simulink model "roll_controller"  (R2021b)
settings: Solver=VariableStepAuto  StartTime=0.0  StopTime=10.0  RelTol=1e-3
settings Model: Creator=aoa  LastModifiedBy=aoa

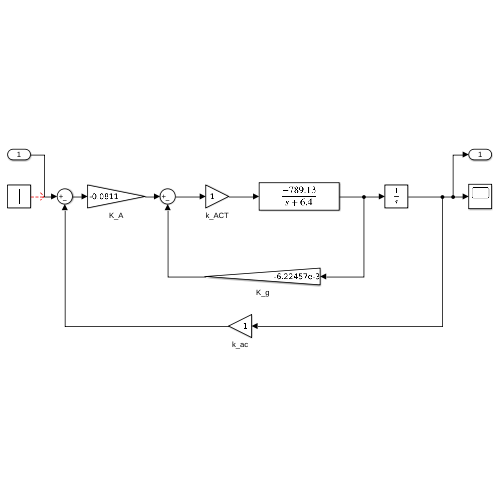
[thumbnail: Simulink's stored preview of the top-level diagram]
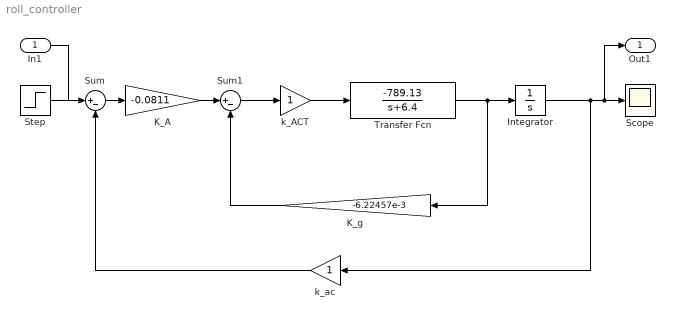
== system roll_controller ==
  In1 : Inport
  Integrator : Integrator
  K_A : Gain  Gain=-0.0811
  K_g : Gain  Gain=-6.22457e-3
  Scope : Scope
  Step : Step  SampleTime=0
  Sum : Sum  Inputs=|+-
  Sum1 : Sum  Inputs=|+-
  Transfer Fcn : TransferFcn  Numerator=[-789.13]  Denominator=[1 6.4]
  k_ACT : Gain
  k_ac : Gain
  Out1 : Outport
  wires:
  Step/1 -> ?
  Sum/1 -> K_A/1
  K_A/1 -> Sum1/1
  Sum1/1 -> k_ACT/1
  k_ACT/1 -> Transfer Fcn/1
  Transfer Fcn/1 -> K_g/1, Integrator/1
  K_g/1 -> Sum1/2
  k_ac/1 -> Sum/2
  Integrator/1 -> k_ac/1, Out1/1, Scope/1
  In1/1 -> Sum/1
